simulink model "Roadsense_ScenarioLibrary"  (R2025b)
settings: Solver=FixedStepDiscrete  StartTime=0.0  StopTime=25  FixedStep=RsTsBase  RelTol=1e-3
undefined symbols (not defined in the file or in its folder): RsTsScenario
settings Model: DataDictionary=Roadsense_Data.sldd  Creator=ragur  LastModifiedBy=ragur

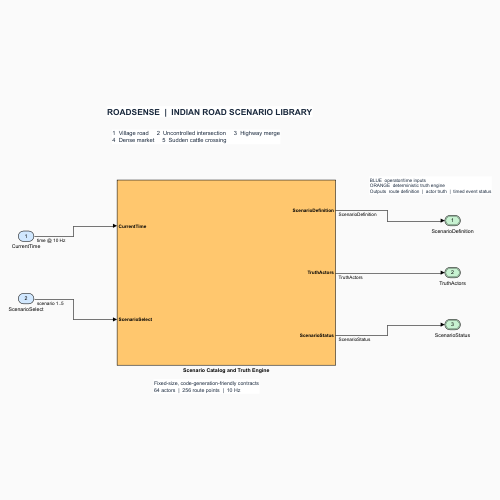
[thumbnail: Simulink's stored preview of the top-level diagram]
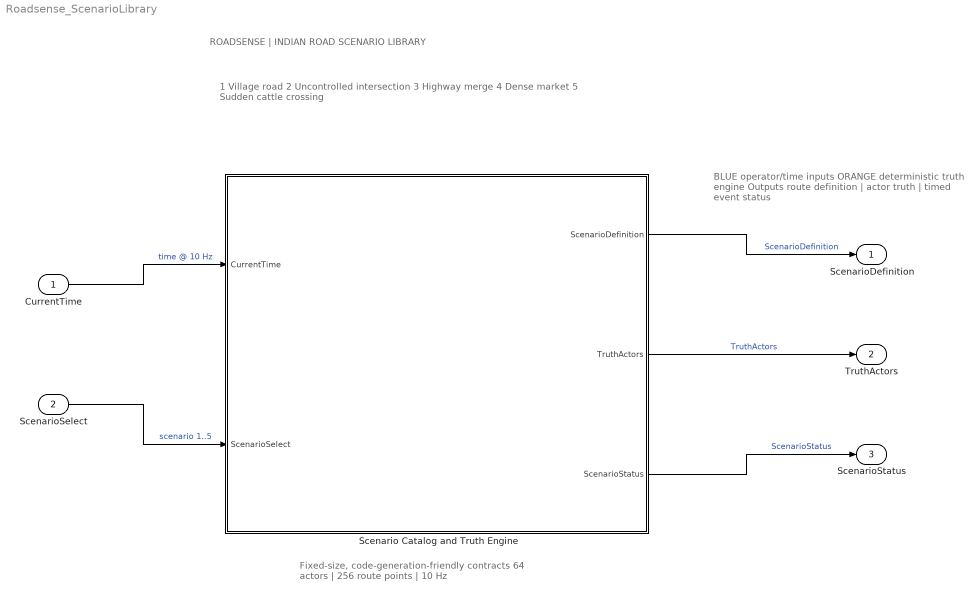
== system Roadsense_ScenarioLibrary ==
  note: ROADSENSE | INDIAN ROAD SCENARIO LIBRARY
  note: 1  Village road     2  Uncontrolled intersection     3  Highway merge
      | 4  Dense market     5  Sudden cattle crossing
  note: BLUE  operator/time inputs
      | ORANGE  deterministic truth engine
      | Outputs  route definition  |  actor truth  |  timed event status
  note: Fixed-size, code-generation-friendly contracts
      | 64 actors  |  256 route points  |  10 Hz
  CurrentTime : Inport  OutDataTypeStr=double  SampleTime=RsTsScenario
  ScenarioSelect : Inport  Port=2  OutDataTypeStr=uint8  SampleTime=RsTsScenario
  Scenario Catalog and Truth Engine : Subsystem
  ScenarioDefinition : Outport  OutDataTypeStr=Bus: RsScenarioDefinitionBus
  TruthActors : Outport  Port=2  OutDataTypeStr=Bus: RsScenarioActorListBus
  ScenarioStatus : Outport  Port=3  OutDataTypeStr=Bus: RsScenarioStatusBus
  wires:
  CurrentTime/1 -> Scenario Catalog and Truth Engine/1(CurrentTime)  "time @ 10 Hz"
  ScenarioSelect/1 -> Scenario Catalog and Truth Engine/2(ScenarioSelect)  "scenario 1..5"
  Scenario Catalog and Truth Engine/1(ScenarioDefinition) -> ScenarioDefinition/1  "ScenarioDefinition"
  Scenario Catalog and Truth Engine/2(TruthActors) -> TruthActors/1  "TruthActors"
  Scenario Catalog and Truth Engine/3(ScenarioStatus) -> ScenarioStatus/1  "ScenarioStatus"

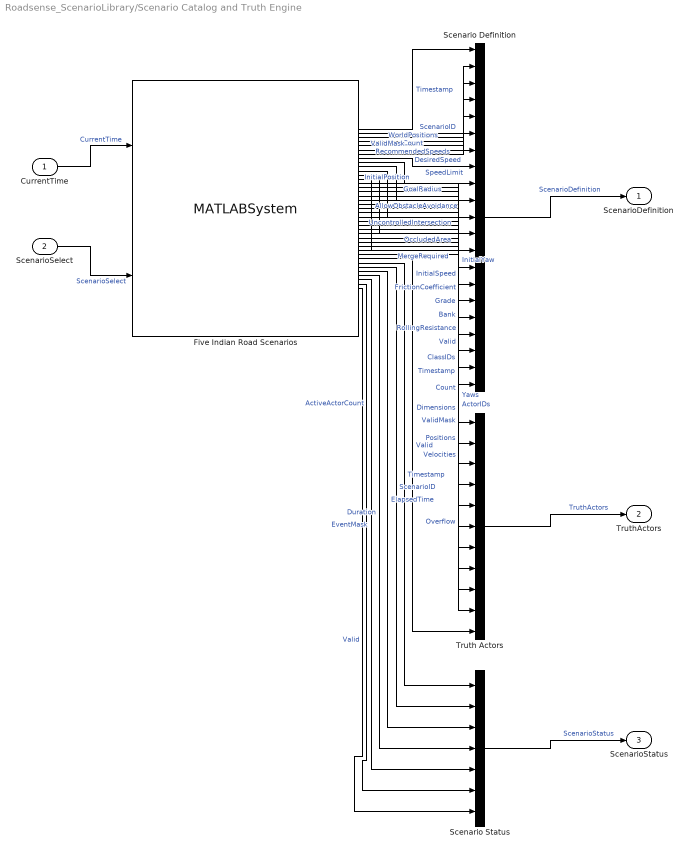
== system Roadsense_ScenarioLibrary/Scenario Catalog and Truth Engine ==
  CurrentTime : Inport  OutDataTypeStr=double
  ScenarioSelect : Inport  Port=2  OutDataTypeStr=uint8
  Five Indian Road Scenarios : MATLABSystem  System=RoadsenseScenarioLibrarySystem  SimulateUsing=Interpreted execution
      mask Type: RoadsenseScenarioLibrarySystem
  Scenario Definition : BusCreator  Inputs=21  OutDataTypeStr=Bus: RsScenarioDefinitionBus
  Scenario Status : BusCreator  Inputs=7  OutDataTypeStr=Bus: RsScenarioStatusBus
  Truth Actors : BusCreator  Inputs=11  OutDataTypeStr=Bus: RsScenarioActorListBus
  ScenarioDefinition : Outport  OutDataTypeStr=Bus: RsScenarioDefinitionBus
  TruthActors : Outport  Port=2  OutDataTypeStr=Bus: RsScenarioActorListBus
  ScenarioStatus : Outport  Port=3  OutDataTypeStr=Bus: RsScenarioStatusBus
  wires:
  CurrentTime/1 -> Five Indian Road Scenarios/1  "CurrentTime"
  ScenarioSelect/1 -> Five Indian Road Scenarios/2  "ScenarioSelect"
  Five Indian Road Scenarios/1 -> Scenario Definition/1  "Timestamp"
  Five Indian Road Scenarios/2 -> Scenario Definition/2  "ScenarioID"
  Five Indian Road Scenarios/3 -> Scenario Definition/3  "Count"
  Five Indian Road Scenarios/4 -> Scenario Definition/4  "WorldPositions"
  Five Indian Road Scenarios/5 -> Scenario Definition/5  "RecommendedSpeeds"
  Five Indian Road Scenarios/6 -> Scenario Definition/6  "ValidMask"
  Five Indian Road Scenarios/7 -> Scenario Definition/7  "DesiredSpeed"
  Five Indian Road Scenarios/8 -> Scenario Definition/8  "SpeedLimit"
  Five Indian Road Scenarios/9 -> Scenario Definition/9  "GoalRadius"
  Five Indian Road Scenarios/10 -> Scenario Definition/10  "AllowObstacleAvoidance"
  Five Indian Road Scenarios/11 -> Scenario Definition/11  "UncontrolledIntersection"
  Five Indian Road Scenarios/12 -> Scenario Definition/12  "OccludedArea"
  Five Indian Road Scenarios/13 -> Scenario Definition/13  "MergeRequired"
  Five Indian Road Scenarios/14 -> Scenario Definition/14  "InitialPosition"
  Five Indian Road Scenarios/15 -> Scenario Definition/15  "InitialYaw"
  Five Indian Road Scenarios/16 -> Scenario Definition/16  "InitialSpeed"
  Five Indian Road Scenarios/17 -> Scenario Definition/17  "FrictionCoefficient"
  Five Indian Road Scenarios/18 -> Scenario Definition/18  "Grade"
  Five Indian Road Scenarios/19 -> Scenario Definition/19  "Bank"
  Five Indian Road Scenarios/20 -> Scenario Definition/20  "RollingResistance"
  Five Indian Road Scenarios/21 -> Scenario Definition/21  "Valid"
  Five Indian Road Scenarios/22 -> Truth Actors/1  "Timestamp"
  Five Indian Road Scenarios/23 -> Truth Actors/2  "Count"
  Five Indian Road Scenarios/24 -> Truth Actors/3  "ActorIDs"
  Five Indian Road Scenarios/25 -> Truth Actors/4  "ClassIDs"
  Five Indian Road Scenarios/26 -> Truth Actors/5  "Positions"
  Five Indian Road Scenarios/27 -> Truth Actors/6  "Velocities"
  Five Indian Road Scenarios/28 -> Truth Actors/7  "Yaws"
  Five Indian Road Scenarios/29 -> Truth Actors/8  "Dimensions"
  Five Indian Road Scenarios/30 -> Truth Actors/9  "ValidMask"
  Five Indian Road Scenarios/31 -> Truth Actors/10  "Overflow"
  Five Indian Road Scenarios/32 -> Truth Actors/11  "Valid"
  Five Indian Road Scenarios/33 -> Scenario Status/1  "Timestamp"
  Five Indian Road Scenarios/34 -> Scenario Status/2  "ScenarioID"
  Five Indian Road Scenarios/35 -> Scenario Status/3  "ElapsedTime"
  Five Indian Road Scenarios/36 -> Scenario Status/4  "Duration"
  Five Indian Road Scenarios/37 -> Scenario Status/5  "EventMask"
  Five Indian Road Scenarios/38 -> Scenario Status/6  "ActiveActorCount"
  Five Indian Road Scenarios/39 -> Scenario Status/7  "Valid"
  Scenario Definition/1 -> ScenarioDefinition/1  "ScenarioDefinition"
  Truth Actors/1 -> TruthActors/1  "TruthActors"
  Scenario Status/1 -> ScenarioStatus/1  "ScenarioStatus"
